simulink subsystem "controller_ref_subsys"  (R2022b)
settings: Solver=VariableStepAuto  StartTime=0.0  StopTime=10.0  RelTol=1e-3
undefined symbols (not defined in the file): param_EKF
settings Model: Creator=emu  LastModifiedBy=rslstudent

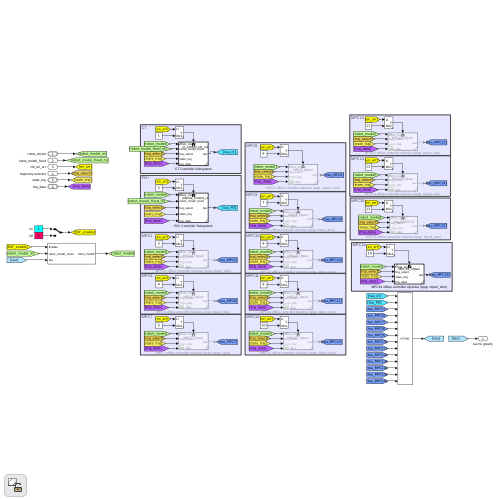
[thumbnail: Simulink's stored preview of the top-level diagram]
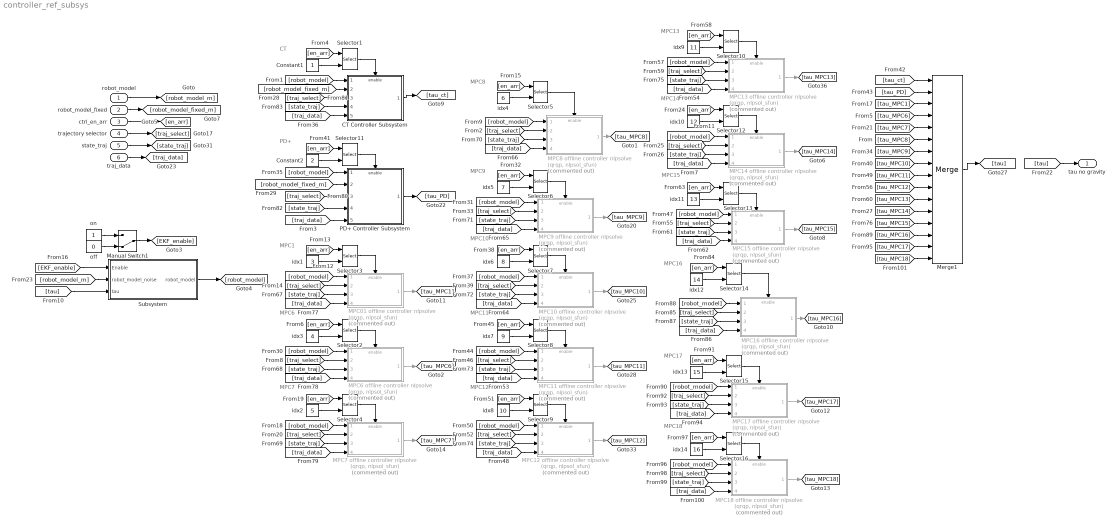
== system controller_ref_subsys ==
  note: MPC15
  note: MPC6
  note: MPC1
  note: CT
  note: MPC7
  note: MPC8
  note: MPC9
  note: MPC10
  note: MPC11
  note: MPC12
  note: MPC13
  note: PD+
  note: MPC14
  note: MPC16
  note: MPC17
  note: MPC18
  robot_model : Inport  OutDataTypeStr=Bus: robot_model
  robot_model_fixed : Inport  Port=2
  ctrl_en_arr : Inport  Port=3
  trajectory selector : Inport  Port=4
  state_traj : Inport  Port=5  OutDataTypeStr=Bus: state_traj_bus
  traj_data : Inport  Port=6  OutDataTypeStr=Bus: traj_data_bus
  CT Controller Subsystem : Subsystem  ReferencedSubsystem=ct_control_ref_subsys
  Constant1 : Constant
  Constant2 : Constant  Value=2
  "MPC01 offline controller nlpsolve (qrqp, nlpsol_sfun)" : Subsystem  Commented=on  ReferencedSubsystem=MPC01_nlpsol
  "MPC10 offline controller nlpsolve (qrqp, nlpsol_sfun)" : Subsystem  Commented=on  ReferencedSubsystem=MPC10_nlpsol
  "MPC11 offline controller nlpsolve (qrqp, nlpsol_sfun)" : Subsystem  Commented=on  ReferencedSubsystem=MPC11_nlpsol
  "MPC12 offline controller nlpsolve (qrqp, nlpsol_sfun)" : Subsystem  Commented=on  ReferencedSubsystem=MPC12_nlpsol
  "MPC13 offline controller nlpsolve (qrqp, nlpsol_sfun)" : Subsystem  Commented=on  ReferencedSubsystem=MPC13_nlpsol
  "MPC14 offline controller nlpsolve (qrqp, nlpsol_sfun)" : Subsystem  Commented=on  ReferencedSubsystem=MPC14_nlpsol
  "MPC15 offline controller nlpsolve (qrqp, nlpsol_sfun)" : Subsystem  Commented=on  ReferencedSubsystem=BilayerMPC15
  "MPC16 offline controller nlpsolve (qrqp, nlpsol_sfun)" : Subsystem  Commented=on  ReferencedSubsystem=MPC16_nlpsol
  "MPC17 offline controller nlpsolve (qrqp, nlpsol_sfun)" : Subsystem  Commented=on  ReferencedSubsystem=MPC17_nlpsol
  "MPC18 offline controller nlpsolve (qrqp, nlpsol_sfun)" : Subsystem  Commented=on  ReferencedSubsystem=MPC01_nlpsol
  "MPC6 offline controller nlpsolve (qrqp, nlpsol_sfun)" : Subsystem  Commented=on  ReferencedSubsystem=MPC6_nlpsol
  "MPC7 offline controller nlpsolve (qrqp, nlpsol_sfun)" : Subsystem  Commented=on  ReferencedSubsystem=MPC7_nlpsol
  "MPC8 offline controller nlpsolve (qrqp, nlpsol_sfun)" : Subsystem  Commented=on  ReferencedSubsystem=MPC8_nlpsol
  "MPC9 offline controller nlpsolve (qrqp, nlpsol_sfun)" : Subsystem  Commented=on  ReferencedSubsystem=MPC9_nlpsol
  Manual Switch1 : ManualSwitch  CurrentSetting=0
  Merge1 : Merge  Inputs=16
  PD+ Controller Subsystem : Subsystem  ReferencedSubsystem=pdplus_control_ref_subsys
  Selector{1..16} (16 alike) : Selector  IndexOptions=Index vector (port)  Indices=[1 3]  OutputSizes=1
  Subsystem : Subsystem
  idx1 : Constant  Value=3
  idx10 : Constant  Value=12
  idx11 : Constant  Value=13
  idx12 : Constant  Value=14
  idx13 : Constant  Value=15
  idx14 : Constant  Value=16
  idx2 : Constant  Value=5
  idx3 : Constant  Value=4
  idx4 : Constant  Value=6
  idx5 : Constant  Value=7
  idx6 : Constant  Value=8
  idx7 : Constant  Value=9
  idx8 : Constant  Value=10
  idx9 : Constant  Value=11
  off : Constant  Value=0
  on : Constant
  tau no gravity : Outport
  wires:
  idx1/1 -> Selector3/2
  Selector1/1 -> CT Controller Subsystem/Enable
  "MPC6 offline controller nlpsolve (qrqp, nlpsol_sfun)"/1 -> [tau_MPC6]
  [traj_select] -> "MPC6 offline controller nlpsolve (qrqp, nlpsol_sfun)"/2
  [en_arr] -> Selector2/1
  robot_model/1 -> [robot_model_m]
  Constant1/1 -> Selector1/2
  trajectory selector/1 -> [traj_select]
  Selector3/1 -> "MPC01 offline controller nlpsolve (qrqp, nlpsol_sfun)"/Enable
  "MPC01 offline controller nlpsolve (qrqp, nlpsol_sfun)"/1 -> [tau_MPC1]
  CT Controller Subsystem/1 -> [tau_ct]
  [robot_model] -> "MPC6 offline controller nlpsolve (qrqp, nlpsol_sfun)"/1
  idx3/1 -> Selector2/2
  Selector2/1 -> "MPC6 offline controller nlpsolve (qrqp, nlpsol_sfun)"/Enable
  [en_arr] -> Selector3/1
  [traj_select] -> "MPC01 offline controller nlpsolve (qrqp, nlpsol_sfun)"/2
  [robot_model] -> "MPC01 offline controller nlpsolve (qrqp, nlpsol_sfun)"/1
  [en_arr] -> Selector1/1
  idx2/1 -> Selector4/2
  Selector4/1 -> "MPC7 offline controller nlpsolve (qrqp, nlpsol_sfun)"/Enable
  [en_arr] -> Selector4/1
  "MPC7 offline controller nlpsolve (qrqp, nlpsol_sfun)"/1 -> [tau_MPC7]
  [traj_select] -> "MPC7 offline controller nlpsolve (qrqp, nlpsol_sfun)"/2
  [robot_model] -> "MPC7 offline controller nlpsolve (qrqp, nlpsol_sfun)"/1
  ctrl_en_arr/1 -> [en_arr]
  "MPC8 offline controller nlpsolve (qrqp, nlpsol_sfun)"/1 -> [tau_MPC8]
  idx5/1 -> Selector6/2
  [traj_select] -> "MPC9 offline controller nlpsolve (qrqp, nlpsol_sfun)"/2
  [en_arr] -> Selector6/1
  Selector6/1 -> "MPC9 offline controller nlpsolve (qrqp, nlpsol_sfun)"/Enable
  "MPC9 offline controller nlpsolve (qrqp, nlpsol_sfun)"/1 -> [tau_MPC9]
  [robot_model] -> "MPC9 offline controller nlpsolve (qrqp, nlpsol_sfun)"/1
  [en_arr] -> Selector7/1
  [traj_select] -> "MPC10 offline controller nlpsolve (qrqp, nlpsol_sfun)"/2
  "MPC10 offline controller nlpsolve (qrqp, nlpsol_sfun)"/1 -> [tau_MPC10]
  Selector7/1 -> "MPC10 offline controller nlpsolve (qrqp, nlpsol_sfun)"/Enable
  [robot_model] -> "MPC10 offline controller nlpsolve (qrqp, nlpsol_sfun)"/1
  idx6/1 -> Selector7/2
  [robot_model] -> "MPC11 offline controller nlpsolve (qrqp, nlpsol_sfun)"/1
  [en_arr] -> Selector8/1
  [traj_select] -> "MPC11 offline controller nlpsolve (qrqp, nlpsol_sfun)"/2
  idx7/1 -> Selector8/2
  "MPC11 offline controller nlpsolve (qrqp, nlpsol_sfun)"/1 -> [tau_MPC11]
  Selector8/1 -> "MPC11 offline controller nlpsolve (qrqp, nlpsol_sfun)"/Enable
  Selector9/1 -> "MPC12 offline controller nlpsolve (qrqp, nlpsol_sfun)"/Enable
  [en_arr] -> Selector9/1
  idx8/1 -> Selector9/2
  [robot_model] -> "MPC12 offline controller nlpsolve (qrqp, nlpsol_sfun)"/1
  "MPC12 offline controller nlpsolve (qrqp, nlpsol_sfun)"/1 -> [tau_MPC12]
  [traj_select] -> "MPC12 offline controller nlpsolve (qrqp, nlpsol_sfun)"/2
  "MPC13 offline controller nlpsolve (qrqp, nlpsol_sfun)"/1 -> [tau_MPC13]
  [en_arr] -> Selector10/1
  [traj_select] -> "MPC13 offline controller nlpsolve (qrqp, nlpsol_sfun)"/2
  idx9/1 -> Selector10/2
  [robot_model] -> "MPC13 offline controller nlpsolve (qrqp, nlpsol_sfun)"/1
  Selector10/1 -> "MPC13 offline controller nlpsolve (qrqp, nlpsol_sfun)"/Enable
  [en_arr] -> Selector5/1
  Selector5/1 -> "MPC8 offline controller nlpsolve (qrqp, nlpsol_sfun)"/Enable
  idx4/1 -> Selector5/2
  [traj_select] -> "MPC8 offline controller nlpsolve (qrqp, nlpsol_sfun)"/2
  [robot_model] -> "MPC8 offline controller nlpsolve (qrqp, nlpsol_sfun)"/1
  [en_arr] -> Selector11/1
  PD+ Controller Subsystem/1 -> [tau_PD]
  Constant2/1 -> Selector11/2
  [robot_model] -> PD+ Controller Subsystem/1
  Selector11/1 -> PD+ Controller Subsystem/Enable
  Merge1/1 -> [tau]
  [state_traj] -> "MPC01 offline controller nlpsolve (qrqp, nlpsol_sfun)"/3
  state_traj/1 -> [state_traj]
  [state_traj] -> "MPC6 offline controller nlpsolve (qrqp, nlpsol_sfun)"/3
  [state_traj] -> "MPC7 offline controller nlpsolve (qrqp, nlpsol_sfun)"/3
  [state_traj] -> "MPC8 offline controller nlpsolve (qrqp, nlpsol_sfun)"/3
  [state_traj] -> "MPC9 offline controller nlpsolve (qrqp, nlpsol_sfun)"/3
  [state_traj] -> "MPC10 offline controller nlpsolve (qrqp, nlpsol_sfun)"/3
  [state_traj] -> "MPC11 offline controller nlpsolve (qrqp, nlpsol_sfun)"/3
  [state_traj] -> "MPC12 offline controller nlpsolve (qrqp, nlpsol_sfun)"/3
  [state_traj] -> "MPC13 offline controller nlpsolve (qrqp, nlpsol_sfun)"/3
  [tau] -> tau no gravity/1
  [tau_MPC8] -> Merge1/6
  [tau_MPC9] -> Merge1/7
  [tau_MPC10] -> Merge1/8
  [tau_MPC11] -> Merge1/9
  [tau_MPC12] -> Merge1/10
  [tau_MPC13] -> Merge1/11
  [tau_MPC1] -> Merge1/3
  [tau_PD] -> Merge1/2
  [tau_ct] -> Merge1/1
  [tau_MPC6] -> Merge1/4
  [tau_MPC7] -> Merge1/5
  [traj_data] -> "MPC12 offline controller nlpsolve (qrqp, nlpsol_sfun)"/4
  [traj_data] -> "MPC11 offline controller nlpsolve (qrqp, nlpsol_sfun)"/4
  [traj_data] -> "MPC9 offline controller nlpsolve (qrqp, nlpsol_sfun)"/4
  [traj_data] -> "MPC8 offline controller nlpsolve (qrqp, nlpsol_sfun)"/4
  [traj_data] -> "MPC01 offline controller nlpsolve (qrqp, nlpsol_sfun)"/4
  [traj_data] -> "MPC6 offline controller nlpsolve (qrqp, nlpsol_sfun)"/4
  [traj_data] -> "MPC7 offline controller nlpsolve (qrqp, nlpsol_sfun)"/4
  [traj_data] -> "MPC10 offline controller nlpsolve (qrqp, nlpsol_sfun)"/4
  [traj_data] -> PD+ Controller Subsystem/5
  [traj_select] -> PD+ Controller Subsystem/3
  [state_traj] -> PD+ Controller Subsystem/4
  [traj_data] -> CT Controller Subsystem/5
  [robot_model] -> CT Controller Subsystem/1
  [traj_data] -> "MPC13 offline controller nlpsolve (qrqp, nlpsol_sfun)"/4
  [state_traj] -> CT Controller Subsystem/4
  [traj_select] -> CT Controller Subsystem/3
  traj_data/1 -> [traj_data]
  on/1 -> Manual Switch1/1
  off/1 -> Manual Switch1/2
  Manual Switch1/1 -> [EKF_enable]
  [EKF_enable] -> Subsystem/1(Enable)
  [robot_model_m] -> Subsystem/2(robot_model_noise)
  [tau] -> Subsystem/3(tau)
  Subsystem/1(robot_model) -> [robot_model]
  [traj_data] -> "MPC14 offline controller nlpsolve (qrqp, nlpsol_sfun)"/4
  [state_traj] -> "MPC14 offline controller nlpsolve (qrqp, nlpsol_sfun)"/3
  Selector12/1 -> "MPC14 offline controller nlpsolve (qrqp, nlpsol_sfun)"/Enable
  [robot_model] -> "MPC14 offline controller nlpsolve (qrqp, nlpsol_sfun)"/1
  idx10/1 -> Selector12/2
  [traj_select] -> "MPC14 offline controller nlpsolve (qrqp, nlpsol_sfun)"/2
  [en_arr] -> Selector12/1
  "MPC14 offline controller nlpsolve (qrqp, nlpsol_sfun)"/1 -> [tau_MPC14]
  [tau_MPC14] -> Merge1/12
  robot_model_fixed/1 -> [robot_model_fixed_m]
  [robot_model_fixed_m] -> CT Controller Subsystem/2
  [robot_model_fixed_m] -> PD+ Controller Subsystem/2
  [robot_model] -> "MPC15 offline controller nlpsolve (qrqp, nlpsol_sfun)"/1
  [traj_select] -> "MPC15 offline controller nlpsolve (qrqp, nlpsol_sfun)"/2
  [state_traj] -> "MPC15 offline controller nlpsolve (qrqp, nlpsol_sfun)"/3
  [traj_data] -> "MPC15 offline controller nlpsolve (qrqp, nlpsol_sfun)"/4
  [en_arr] -> Selector13/1
  idx11/1 -> Selector13/2
  Selector13/1 -> "MPC15 offline controller nlpsolve (qrqp, nlpsol_sfun)"/Enable
  "MPC15 offline controller nlpsolve (qrqp, nlpsol_sfun)"/1 -> [tau_MPC15]
  [tau_MPC15] -> Merge1/13
  [traj_data] -> "MPC16 offline controller nlpsolve (qrqp, nlpsol_sfun)"/4
  [state_traj] -> "MPC16 offline controller nlpsolve (qrqp, nlpsol_sfun)"/3
  [robot_model] -> "MPC16 offline controller nlpsolve (qrqp, nlpsol_sfun)"/1
  [traj_select] -> "MPC16 offline controller nlpsolve (qrqp, nlpsol_sfun)"/2
  idx12/1 -> Selector14/2
  Selector14/1 -> "MPC16 offline controller nlpsolve (qrqp, nlpsol_sfun)"/Enable
  [en_arr] -> Selector14/1
  "MPC16 offline controller nlpsolve (qrqp, nlpsol_sfun)"/1 -> [tau_MPC16]
  [tau_MPC16] -> Merge1/14
  [traj_data] -> "MPC17 offline controller nlpsolve (qrqp, nlpsol_sfun)"/4
  [state_traj] -> "MPC17 offline controller nlpsolve (qrqp, nlpsol_sfun)"/3
  [robot_model] -> "MPC17 offline controller nlpsolve (qrqp, nlpsol_sfun)"/1
  [traj_select] -> "MPC17 offline controller nlpsolve (qrqp, nlpsol_sfun)"/2
  [en_arr] -> Selector15/1
  "MPC17 offline controller nlpsolve (qrqp, nlpsol_sfun)"/1 -> [tau_MPC17]
  Selector15/1 -> "MPC17 offline controller nlpsolve (qrqp, nlpsol_sfun)"/Enable
  idx13/1 -> Selector15/2
  [tau_MPC17] -> Merge1/15
  idx14/1 -> Selector16/2
  Selector16/1 -> "MPC18 offline controller nlpsolve (qrqp, nlpsol_sfun)"/Enable
  "MPC18 offline controller nlpsolve (qrqp, nlpsol_sfun)"/1 -> [tau_MPC18]
  [en_arr] -> Selector16/1
  [traj_select] -> "MPC18 offline controller nlpsolve (qrqp, nlpsol_sfun)"/2
  [robot_model] -> "MPC18 offline controller nlpsolve (qrqp, nlpsol_sfun)"/1
  [state_traj] -> "MPC18 offline controller nlpsolve (qrqp, nlpsol_sfun)"/3
  [traj_data] -> "MPC18 offline controller nlpsolve (qrqp, nlpsol_sfun)"/4
  [tau_MPC18] -> Merge1/16

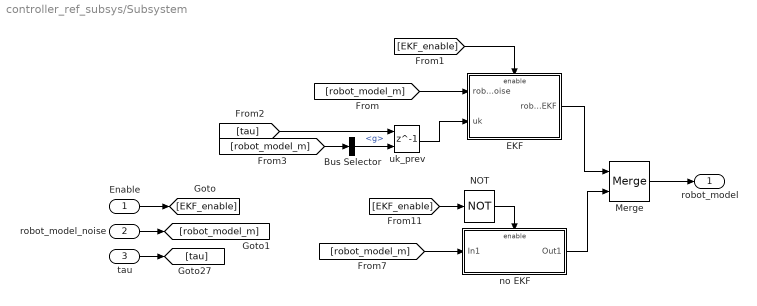
== system controller_ref_subsys/Subsystem ==
  Enable : Inport
  robot_model_noise : Inport  Port=2  OutDataTypeStr=Bus: robot_model
  tau : Inport  Port=3
  Bus Selector : BusSelector  OutputSignals=g
  EKF : Subsystem
  Merge : Merge
  NOT : Logic  Operator=NOT  IconShape=distinctive  AllPortsSameDT=off  OutDataTypeStr=boolean
  no EKF : Subsystem
  uk_prev : Delay  DelayLength=1  InitialConditionSource=Input port
      settings: InputPortMap=u0,p4
  robot_model : Outport  OutDataTypeStr=Bus: robot_model
  wires:
  [robot_model_m] -> Bus Selector/1
  [tau] -> uk_prev/1
  tau/1 -> [tau]
  robot_model_noise/1 -> [robot_model_m]
  Enable/1 -> [EKF_enable]
  [EKF_enable] -> EKF/Enable
  NOT/1 -> no EKF/Enable
  EKF/1(robot_model_EKF) -> Merge/1
  [robot_model_m] -> EKF/1(robot_model_noise)
  Bus Selector/1 -> uk_prev/2  "<g>"
  Merge/1 -> robot_model/1
  [EKF_enable] -> NOT/1
  uk_prev/1 -> EKF/2(uk)
  no EKF/1(Out1) -> Merge/2
  [robot_model_m] -> no EKF/1(In1)

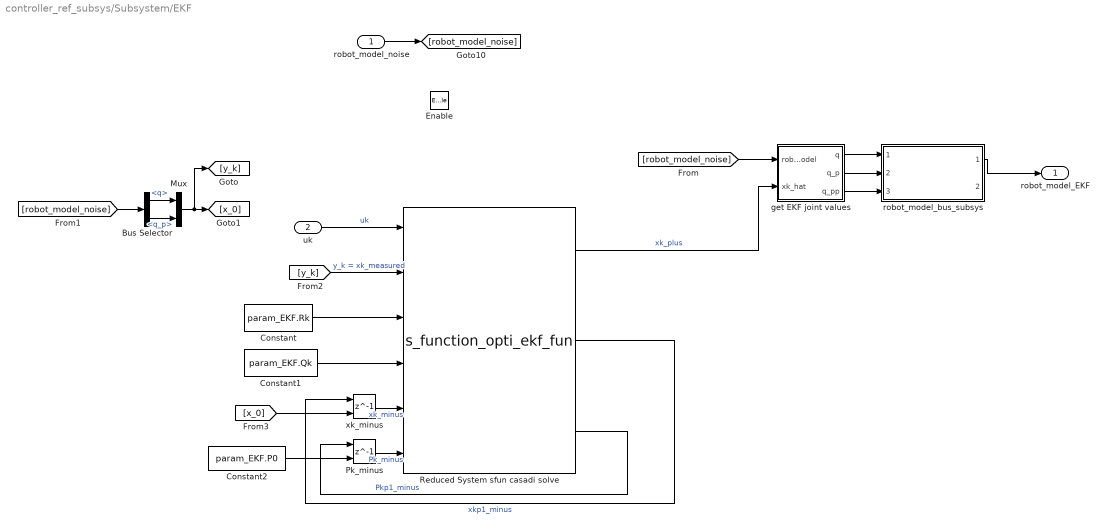
== system controller_ref_subsys/Subsystem/EKF ==
  robot_model_noise : Inport  OutDataTypeStr=Bus: robot_model
  uk : Inport  Port=2
  Enable : EnablePort
  Bus Selector : BusSelector  OutputSignals=q,q_p
  Constant : Constant  Value=param_EKF.Rk
  Constant1 : Constant  Value=param_EKF.Qk
  Constant2 : Constant  Value=param_EKF.P0
  Mux : Mux  Inputs=2
  Pk_minus : Delay  DelayLength=1  InitialConditionSource=Input port
      settings: InputPortMap=u0,p4
  Reduced System sfun casadi solve : S-Function  FunctionName=s_function_opti_ekf_fun  SFunctionModules='ekf_fun'  SFunctionDeploymentMode=off  EnableBusSupport=off
  get EKF joint values : MATLAB Function  TreatAsAtomicUnit=on
  robot_model_bus_subsys : Subsystem  ReferencedSubsystem=robot_model_bus_7dof_ref_subsys
  xk_minus : Delay  DelayLength=1  InitialConditionSource=Input port
      settings: InputPortMap=u0,p4
  robot_model_EKF : Outport  OutDataTypeStr=Bus: robot_model
  wires:
  Mux/1 -> [x_0], [y_k]
  Bus Selector/2 -> Mux/2  "<q_p>"
  Bus Selector/1 -> Mux/1  "<q>"
  Constant2/1 -> Pk_minus/2
  robot_model_bus_subsys/1 -> robot_model_EKF/1
  get EKF joint values/1(q) -> robot_model_bus_subsys/1
  get EKF joint values/2(q_p) -> robot_model_bus_subsys/2
  get EKF joint values/3(q_pp) -> robot_model_bus_subsys/3
  [x_0] -> xk_minus/2
  [y_k] -> Reduced System sfun casadi solve/2  "y_k = xk_measured"
  [robot_model_noise] -> get EKF joint values/1(robot_model)
  Reduced System sfun casadi solve/1 -> get EKF joint values/2(xk_hat)  "xk_plus"
  [robot_model_noise] -> Bus Selector/1
  robot_model_noise/1 -> [robot_model_noise]
  Reduced System sfun casadi solve/2 -> xk_minus/1  "xkp1_minus"
  Reduced System sfun casadi solve/3 -> Pk_minus/1  "Pkp1_minus"
  Pk_minus/1 -> Reduced System sfun casadi solve/6  "Pk_minus"
  xk_minus/1 -> Reduced System sfun casadi solve/5  "xk_minus"
  Constant/1 -> Reduced System sfun casadi solve/3
  Constant1/1 -> Reduced System sfun casadi solve/4
  uk/1 -> Reduced System sfun casadi solve/1  "uk"

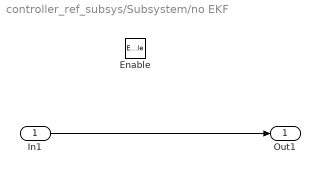
== system controller_ref_subsys/Subsystem/no EKF ==
  In1 : Inport
  Enable : EnablePort
  Out1 : Outport
  wires:
  In1/1 -> Out1/1

== matlab function controller_ref_subsys/Subsystem/EKF/get EKF joint values ==
  data: robot_model input Bus: robot_model; q output; xk_hat input; q_p output; q_pp output; param_robot parameter
function [q, q_p, q_pp] = fcn(robot_model, xk_hat, param_robot)

n_DOF = param_robot.n_DOF;

q = xk_hat(1:n_DOF);
q_p = xk_hat(n_DOF+1:2*n_DOF);
q_pp = robot_model.q_pp;
